simulink model "questao5_simulink"  (R2022b)
settings: Solver=VariableStepAuto  StartTime=0.0  StopTime=0.1  RelTol=1e-3
model workspace (MAT data in the model file):
  C = 0.0008
  L = 0.001
  R = 1
  Vi = 1
  f = 2000
  pid = 5
libraries: slpidlib x1, simulink x1
settings Model: Creator=pedro  LastModifiedBy=maria

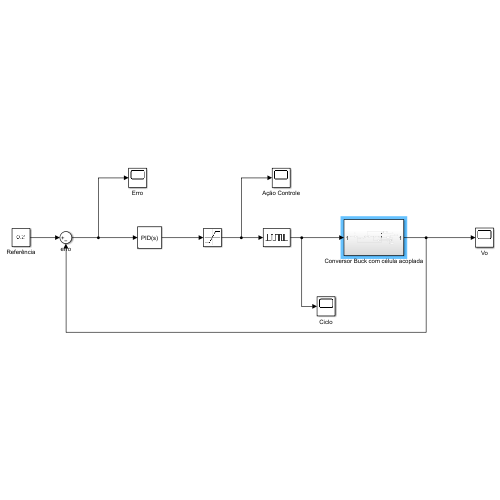
[thumbnail: Simulink's stored preview of the top-level diagram]
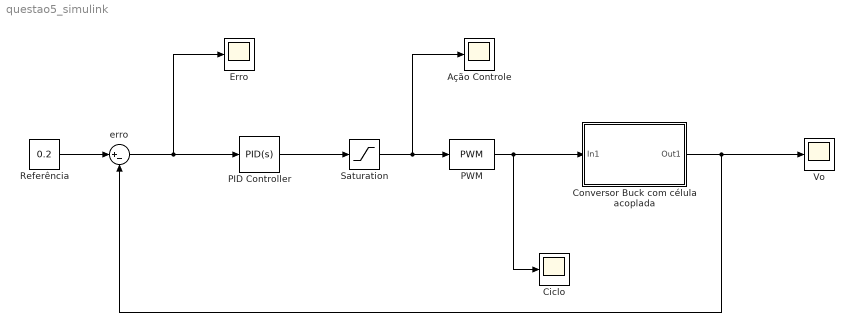
== system questao5_simulink ==
  Ação Controle : Scope
  Ciclo : Scope
  Conversor Buck com célula acoplada : Subsystem
  Erro : Scope
  PID Controller : slpidlib/PID Controller  Controller=PID  Form=Parallel  TimeDomain=Continuous-time  UseExternalTs=off  SampleTime=-1  IntegratorMethod=Forward Euler  FilterMethod=Forward Euler  ControllerParametersSource=internal  P=0.05  I=0  UseKiTs=off  D=0.005  N=1  UseFilter=on  TunerSelectOption=Frequency Response Based  InitialConditionSource=internal  InitialConditionForIntegrator=0.2  InitialConditionForFilter=0  DifferentiatorICPrevScaledInput=0  ExternalReset=none  TrackingMode=off  Kt=1  LimitOutput=off  SatLimitsSource=internal  UpperSaturationLimit=inf  LowerSaturationLimit=-inf  LinearizeAsGain=on  AntiWindupMode=none  Kb=1  LimitIntegrator=off  UpperIntegratorSaturationLimit=inf  LowerIntegratorSaturationLimit=-inf  POutMin=[]  POutMax=[]  IOutMin=[]  IOutMax=[]  DOutMin=[]  DOutMax=[]  NOutMin=[]  NOutMax=[]  SumOutMin=[]  SumOutMax=[]  SaturationOutMin=[]  SaturationOutMax=[]  PParamMin=[]  PParamMax=[]  IParamMin=[]  IParamMax=[]  DParamMin=[]  DParamMax=[]  NParamMin=[]  NParamMax=[]  KbParamMin=[]  KbParamMax=[]  KtParamMin=[]  KtParamMax=[]  KbOutMin=[]  KbOutMax=[]  KtOutMin=[]  KtOutMax=[]  IntegratorOutMin=[]  IntegratorOutMax=[]  FilterOutMin=[]  FilterOutMax=[]  SumI1OutMin=[]  SumI1OutMax=[]  SumI2OutMin=[]  SumI2OutMax=[]  SumI3OutMin=[]  SumI3OutMax=[]  SumI4OutMin=[]  SumI4OutMax=[]  SumDOutMin=[]  SumDOutMax=[]  DifferentiatorOutMin=[]  DifferentiatorOutMax=[]  FilterDiffOutCoefMin=[]  FilterDiffOutCoefMax=[]  ReciprocalOutMin=[]  ReciprocalOutMax=[]  SumDenOutMin=[]  SumDenOutMax=[]  SumNumOutMin=[]  SumNumOutMax=[]  DivideOutMin=[]  DivideOutMax=[]  UdiffTsProdOutMin=[]  UdiffTsProdOutMax=[]  NTsProdOutMin=[]  NTsProdOutMax=[]  UintegralTsProdOutMin=[]  UintegralTsProdOutMax=[]  UngainTsProdOutMin=[]  UngainTsProdOutMax=[]  ClampingZeroOutDataTypeStr=Inherit: Inherit via back propagation  ClampingZeroOutMin=[]  ClampingZeroOutMax=[]  FilterDenConstantOutDataTypeStr=Inherit: Inherit via back propagation  FilterDenConstantOutMin=[]  FilterDenConstantOutMax=[]  PCopyOutDataTypeStr=Inherit: Inherit via back propagation  PCopyOutMin=[]  PCopyOutMax=[]  NCopyOutDataTypeStr=Inherit: Inherit via back propagation  NCopyOutMin=[]  NCopyOutMax=[]  IntegratorContinuousStateAttributes=''  IntegratorStateMustResolveToSignalObject=off  IntegratorRTWStateStorageClass=Auto  FilterContinuousStateAttributes=''  FilterStateMustResolveToSignalObject=off  FilterRTWStateStorageClass=Auto  ParallelPVariant=InternalParameters  IdealPVariant=Disabled  IVariant=InternalParameters  DVariant=InternalParameters  IntegratorVariant=Continuous  SatVariant=Disabled  AWVariant=Passthrough  PCopyVariant=Disabled  TRVariant=Disabled  FdbkBlocksVariant=Forward  IdealPFdbkVariant=Disabled  SatFdbkVariant=Disabled  DerivativeFilterVariant=ContFilter  NVariant=InternalParameters  NCopyVariant=Disabled  FilterICVariant=InternalICsFilter  IntegratorICVariant=InternalICs  ExternalResetVariant=Disabled  TRSumVariant=Passthrough  SumFdbkVariant=Disabled  SumVariant=Sum_PID  TsampFilterVariant=InternalTs  TsampNgainVariant=Passthrough  TsampIntegralVariant=Passthrough  ExternalSaturationOutDataTypeStr=Inherit: Same as second input
  PWM : simulink/Discontinuities/PWM  DisableCoverage=on  Period=1/f  InitialDelay=0  DisallowZeroDutyCycle=off  RunAtFixedTimeIntervals=off  SampleTime=0.1
  Referência : Constant  Value=0.2
  Saturation : Saturate  UpperLimit=1  LowerLimit=0
  Vo : Scope
  erro : Sum  Inputs=|+-
  wires:
  Referência/1 -> erro/1
  PWM/1 -> Ciclo/1, Conversor Buck com célula acoplada/1(In1)
  Saturation/1 -> PWM/1, Ação Controle/1
  Conversor Buck com célula acoplada/1(Out1) -> erro/2, Vo/1
  PID Controller/1 -> Saturation/1
  erro/1 -> Erro/1, PID Controller/1

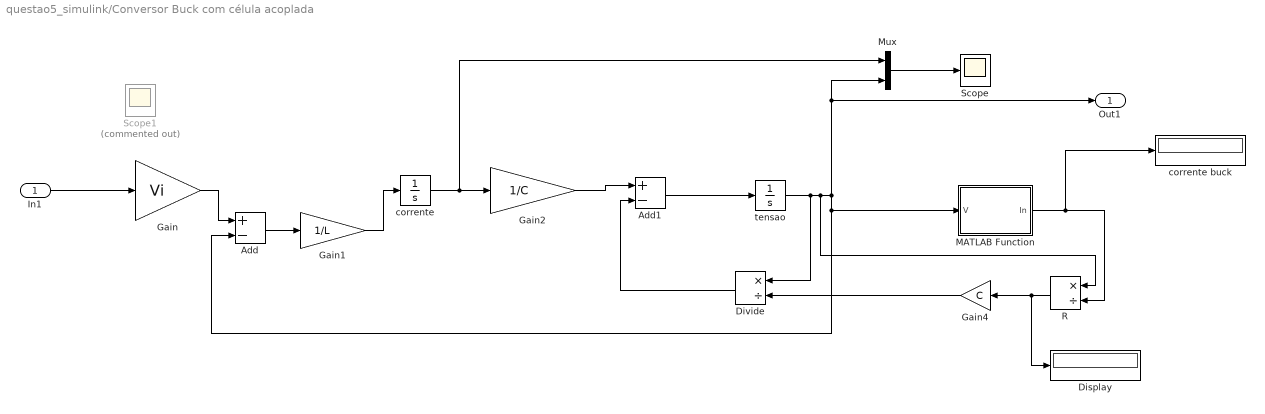
== system questao5_simulink/Conversor Buck com célula acoplada ==
  In1 : Inport
  Add : Sum  Inputs=+-
  Add1 : Sum  Inputs=+-
  Display : Display
  Divide : Product  Inputs=*/  RndMeth=Zero  SaturateOnIntegerOverflow=on
  Gain : Gain  Gain=Vi
  Gain1 : Gain  Gain=1/L
  Gain2 : Gain  Gain=1/C
  Gain4 : Gain  Gain=C
  MATLAB Function : MATLAB Function  TreatAsAtomicUnit=on
  Mux : Mux  Inputs=2
  R : Product  Inputs=*/  RndMeth=Zero  SaturateOnIntegerOverflow=on
  Scope : Scope
  Scope1 : Scope  Commented=on
  corrente : Integrator  InitialCondition=-3.1
  corrente buck : Display
  tensao : Integrator  InitialCondition=0.2
  Out1 : Outport
  wires:
  Divide/1 -> Add1/2
  tensao/1 -> Divide/1, R/1, MATLAB Function/1(V), Add/2, Out1/1, Mux/2
  Gain4/1 -> Divide/2
  MATLAB Function/1(In) -> corrente buck/1, R/2
  In1/1 -> Gain/1
  Gain/1 -> Add/1
  R/1 -> Display/1, Gain4/1
  Gain1/1 -> corrente/1
  Gain2/1 -> Add1/1
  Add/1 -> Gain1/1
  Add1/1 -> tensao/1
  corrente/1 -> Mux/1, Gain2/1
  Mux/1 -> Scope/1

== matlab function questao5_simulink/Conversor Buck com célula acoplada/MATLAB Function ==
  data: V input; In output
function In = resistencia_celula(V)

Gn = 1000; %[W/m^2] irradiação solar nominal
G = Gn; %[W/m^2] irradiação solar
Isen = 3.1656; %[A] corrente de curto-circuito nominal
Ki = 1.8*10^-3; %[A/◦C] coef. de temperatura da corrente de curto-circuito
Tn = 298; %[K] temp. nominal da célula fotovoltaica
Rp = 38.17; %[Ω] resistência paralela (shunt)
A = 1.7538; %fator de idealidade do diodo
Rs = 61.3*10^-3; %[Ω] resistência série
Is = 5.68*10^-6; %[A] corrente de saturação do diodo (valor nominal) 



k = 1.38*10^-23; %[J/K] constante de Boltzmann
q = 1.602*10^-19; %[C] carga do elétron
T = 298; %[K] temperatura da célula

Vt = (k*T)/q;
tol = 0.001;
lambda = 0.3;
In = 0;



var = 10*tol;
iter = 0;
while (abs(var) > tol && iter <= 1000)

    Ia = In;
    
    Ipv = (G/Gn)*(Isen+Ki*(T-Tn));
   
    Id = Is*(exp((V+Rs*Ia)/(Vt*A))-1);
  
    Ip = (V+(Rs*Ia))/Rp;
    
    In = Ipv - Id - Ip;
    In = lambda*In + (1-lambda)*Ia; %corrente da célula
    
    var = In-Ia;
    iter = iter +1;
    
end

In = -In; %corrente do buck
return
